simulink model "Assignment_acm"  (R2019b)
settings: Solver=VariableStepAuto  StartTime=0.0  StopTime=15.0  RelTol=1e-3
libraries: simulink x5, powerlib x4, eePowerMeasurement x1
settings Model: SnapshotBufferSize=20  SnapshotInterval=20  Creator=manda  LastModifiedBy=manda

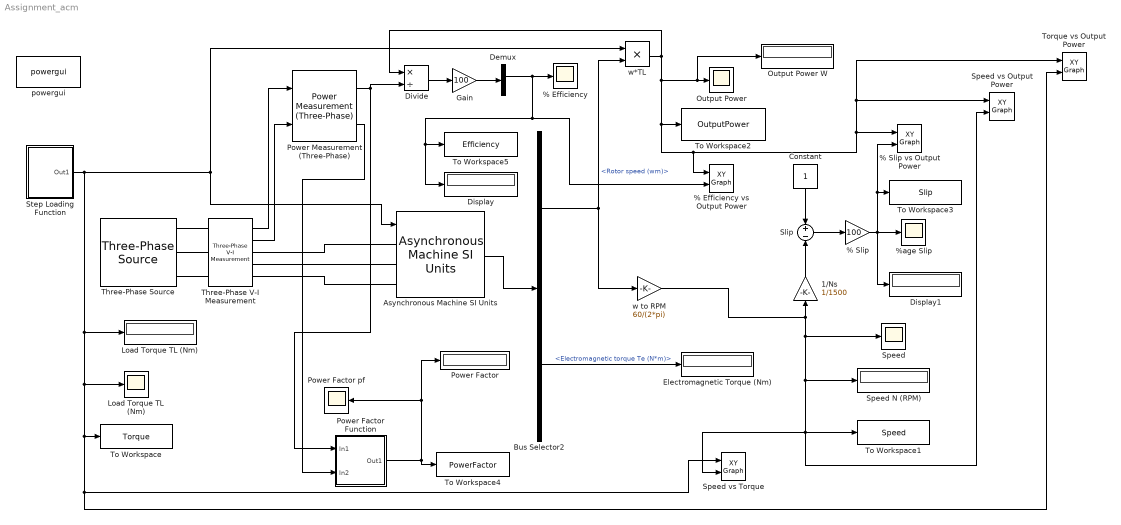
== system Assignment_acm ==
  % Efficiency : Scope
  % Efficiency vs Output Power : simulink/Sinks/XY Graph  xmin=0  xmax=inf  ymin=0  ymax=inf  st=0.1
  % Slip : Gain  Gain=100
  % Slip vs Output Power : simulink/Sinks/XY Graph  xmin=0  xmax=inf  ymin=0  ymax=inf  st=0.1
  %age Slip : Scope
  1/Ns : Gain  Gain=1/1500
  Asynchronous Machine SI Units : powerlib/Machines/Asynchronous Machine SI Units  RotorType=Squirrel-cage  PresetModel=No  MechanicalLoad=Torque Tm  ShowDetailedParameters=on  ReferenceFrame=Rotor  Units=SI  MeasurementBus=off  NominalParameters=[3700 415 50]  Stator=[1.405 0.005839]  Rotor=[1.395 0.005839]  Cage1=[0.4155 0.002066]  Cage2=[0.4168 0.0003495]  Lm=0.1722  Mechanical=[0.0131 0.002985 2]  PolePairs=2  InitialConditions=[0 0 0 0 0 0 0 0]  SimulateSaturation=off  Saturation=[14.03593122, 27.81365428, 53.79336849, 72.68890987, 97.98006896, 148.6815601, 215.7428561, 302.9841135, 428.7778367 ; 230, 322, 414, 460, 506, 552, 598, 644, 690]  LoadFlowParameters=1492000  TsPowergui=0  TsBlock=-1  IterativeModel=Trapezoidal non iterative  IterativeDiscreteModel=Trapezoidal non iterative  Pmec=1.492e+006
      settings: SourceProductName=Simscape Electrical
  Bus Selector2 : BusSelector  OutputSignals=Mechanical.Rotor speed (wm),Mechanical.Electromagnetic torque Te (N*m)
  Constant : Constant
  Demux : Demux
  Display : Display
  Display1 : Display
  Divide : Product  Inputs=*/
  Electromagnetic Torque (Nm) : Display
  Gain : Gain  Gain=100
  Load Torque TL (Nm) : Display
  "Load Torque TL (Nm) " : Scope
  Output Power : Scope
  Output Power W : Display
  Power Factor : Display
  Power Factor Function : Subsystem
  Power Factor pf : Scope
  Power Measurement (Three-Phase) : eePowerMeasurement/Power Measurement (Three-Phase)  LabelModeActiveChoice=Continuous  F=50  K=[0 1 2 3]  Seq=Positive  Ts=0
      settings: SourceProductName=Simscape Electrical  SourceProductBaseCode=PS
  Slip : Sum  Inputs=+-
  Speed : Scope
  Speed N (RPM) : Display
  Speed vs Output Power : simulink/Sinks/XY Graph  xmin=0  xmax=inf  ymin=0  ymax=inf  st=0.1
  Speed vs Torque : simulink/Sinks/XY Graph  xmin=0  xmax=inf  ymin=0  ymax=inf  st=0.1
  Step Loading Function : Subsystem
  Three-Phase V-I Measurement : powerlib/Measurements/Three-Phase V-I Measurement  VoltageMeasurement=phase-to-ground  SetLabelV=off  LabelV=Vabc  Vpu=off  VpuLL=off  CurrentMeasurement=yes  SetLabelI=off  LabelI=Iabc  Ipu=off  Pbase=100e6  Vbase=500e3  OutputType=Complex  PhasorSimulation=off  PSBequivalent=0
      settings: SourceProductName=Simscape Electrical
  Three-Phase Source : powerlib/Electrical Sources/Three-Phase Source  InternalConnection=Yg  VoltagePhases=off  Voltage=415  PhaseAngle=0  Voltage_phases=[25e3 25e3 25e3]/sqrt(3)  PhaseAngles_phases=[0 -120 +120]  Frequency=50  NonIdealSource=off  SpecifyImpedance=off  Resistance=0  Inductance=0  ShortCircuitLevel=100e6  BaseVoltage=25e3  XRratio=7  BusType=swing  Pref=10e3  Qref=0  Prefabc=[10e3, 10e3, 10e3]  Qrefabc=[0, 0, 0]  Qmin=-inf  Qmax=inf
      settings: SourceProductName=Simscape Electrical
  To Workspace : ToWorkspace  VariableName=Torque  SampleTime=0.1
      settings: Decimation=2
  To Workspace1 : ToWorkspace  VariableName=Speed  SampleTime=0.1
      settings: Decimation=2
  To Workspace2 : ToWorkspace  VariableName=OutputPower  SampleTime=0.1
      settings: Decimation=2
  To Workspace3 : ToWorkspace  VariableName=Slip  SampleTime=0.1
      settings: Decimation=2
  To Workspace4 : ToWorkspace  VariableName=PowerFactor  SampleTime=0.1
      settings: Decimation=2
  To Workspace5 : ToWorkspace  VariableName=Efficiency  SampleTime=0.1
      settings: Decimation=2
  Torque vs Output Power : simulink/Sinks/XY Graph  xmin=0  xmax=inf  ymin=0  ymax=inf  st=0.1
  powergui : powerlib/powergui  Priority=1  SimulationMode=Continuous  SampleTime=50e-6  frequency=60  Iterations=50  frequencyindice=50  Pbase=100e6  ErrMax=1e-4  UnitsV=kV  UnitsW=MW  buscounter=0  FunctionMessages=off  echomessages=off  EnableUseOfTLC=off  CurrentSourceSwitches=off  DisableSnubberDevices=off  DisableRonSwitches=off  DisableVfSwitches=off  DisplayEquations=off  AutomaticDiscreteSolvers=off  SolverType=Tustin/Backward Euler (TBE)  Interpol=off  ExternalGateDelay=off  methode=off  Ts=100  x0status=blocks  SPID=on  SwTol=0  HookPort=off  NonlinearTolerance=1e-4  nMaxIteration=100  ContinueOnMaxIteration=off  RestoreLinks=warning  ResistiveCurrentMeasurement=off  Frange=[0:2:500]  Ylog=off  Xlog=on  ShowGrid=off  save=off  variable=ZData  structure=0  ZoomFFT=off  StartTime=0.0  cycles=1  DisplayStyle=1  fundamental=60  FreqAxis=off  MaxFrequency=1000  frequencyindicesteady=1  RmsSteady=1  display=off
      settings: SourceProductName=Simscape Electrical
  w to RPM : Gain  Gain=60/(2*pi)
  w*TL : Product
  wires:
  Asynchronous Machine SI Units/1 -> Bus Selector2/1
  Bus Selector2/1 -> w*TL/2, w to RPM/1  "<Rotor speed (wm)>"
  Bus Selector2/2 -> Electromagnetic Torque (Nm)/1  "<Electromagnetic torque Te (N*m)>"
  w to RPM/1 -> Speed/1, Speed N (RPM)/1, To Workspace1/1, Speed vs Output Power/2, Speed vs Torque/2, 1/Ns/1
  Step Loading Function/1(Out1) -> Torque vs Output Power/2, Speed vs Torque/1, To Workspace/1, "Load Torque TL (Nm) "/1, Load Torque TL (Nm)/1, Asynchronous Machine SI Units/1, w*TL/1
  Constant/1 -> Slip/1
  1/Ns/1 -> Slip/2
  Slip/1 -> % Slip/1
  w*TL/1 -> Divide/1, % Efficiency vs Output Power/1, % Slip vs Output Power/1, Speed vs Output Power/1, Torque vs Output Power/1, To Workspace2/1, Output Power W/1, Output Power/1
  % Slip/1 -> Display1/1, %age Slip/1, % Slip vs Output Power/2, To Workspace3/1
  Power Measurement (Three-Phase)/1 -> Divide/2, Power Factor Function/1(In1)
  Power Measurement (Three-Phase)/2 -> Power Factor Function/2(In2)
  Power Factor Function/1(Out1) -> Power Factor pf/1, Power Factor/1, To Workspace4/1
  Three-Phase V-I Measurement/1 -> Power Measurement (Three-Phase)/1
  Three-Phase V-I Measurement/2 -> Power Measurement (Three-Phase)/2
  Divide/1 -> Gain/1
  Gain/1 -> Demux/1
  Demux/2 -> % Efficiency/1, % Efficiency vs Output Power/2, Display/1, To Workspace5/1
  connections:
  Three-Phase V-I Measurement/LConn1 -- Three-Phase Source/RConn1
  Three-Phase V-I Measurement/LConn2 -- Three-Phase Source/RConn2
  Three-Phase V-I Measurement/RConn1 -- Asynchronous Machine SI Units/LConn1
  Three-Phase V-I Measurement/RConn2 -- Asynchronous Machine SI Units/LConn2
  Three-Phase V-I Measurement/RConn3 -- Asynchronous Machine SI Units/LConn3
  Three-Phase V-I Measurement/LConn3 -- Three-Phase Source/RConn3

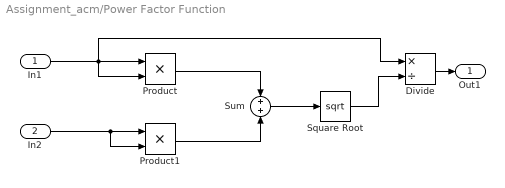
== system Assignment_acm/Power Factor Function ==
  In1 : Inport
  In2 : Inport  Port=2
  Divide : Product  Inputs=*/
  Product : Product
  Product1 : Product
  Square Root : Sqrt  SaturateOnIntegerOverflow=on
  Sum : Sum
  Out1 : Outport
  wires:
  Product1/1 -> Sum/2
  Product/1 -> Sum/1
  Sum/1 -> Square Root/1
  In2/1 -> Product1/2, Product1/1
  Square Root/1 -> Divide/2
  In1/1 -> Product/2, Divide/1, Product/1
  Divide/1 -> Out1/1

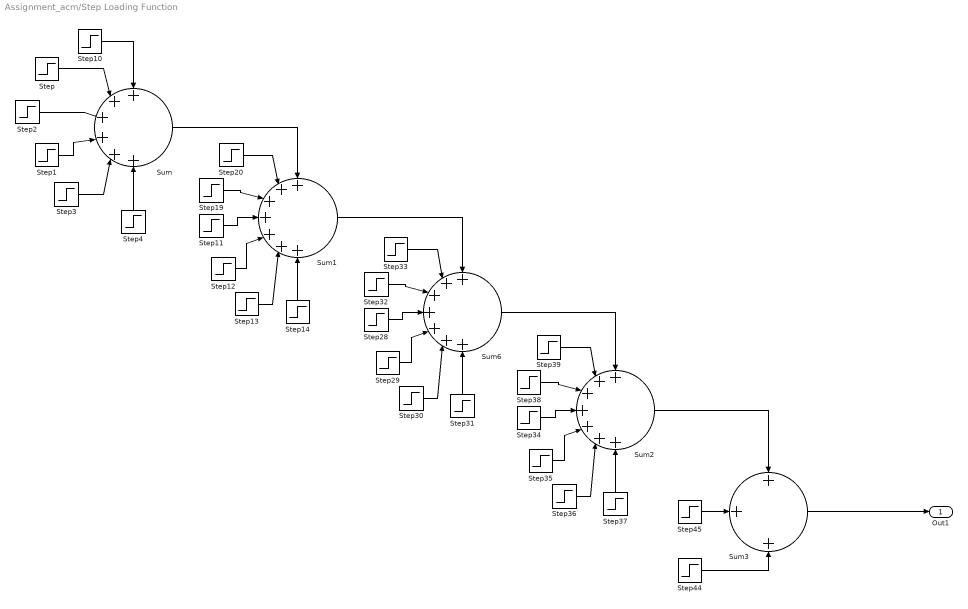
== system Assignment_acm/Step Loading Function ==
  Step : Step  Time=1.5  After=1.23  SampleTime=0
  Step1 : Step  Time=2.5  After=1.23  SampleTime=0
  Step10 : Step  After=1.23  SampleTime=0
  Step11 : Step  Time=5  After=1.23  SampleTime=0
  Step12 : Step  Time=5.5  After=1.23  SampleTime=0
  Step13 : Step  Time=6  After=1.23  SampleTime=0
  Step14 : Step  Time=6.5  After=1.23  SampleTime=0
  Step19 : Step  Time=4.5  After=1.23  SampleTime=0
  Step2 : Step  Time=2  After=1.23  SampleTime=0
  Step20 : Step  Time=4  After=1.23  SampleTime=0
  Step28 : Step  Time=8  After=1.23  SampleTime=0
  Step29 : Step  Time=8.5  After=1.23  SampleTime=0
  Step3 : Step  Time=3  After=1.23  SampleTime=0
  Step30 : Step  Time=9  After=1.23  SampleTime=0
  Step31 : Step  Time=9.5  After=1.23  SampleTime=0
  Step32 : Step  Time=7.5  After=1.23  SampleTime=0
  Step33 : Step  Time=7  After=1.23  SampleTime=0
  Step34 : Step  Time=11  After=1.23  SampleTime=0
  Step35 : Step  Time=11.5  After=1.23  SampleTime=0
  Step36 : Step  Time=12  After=1.23  SampleTime=0
  Step37 : Step  Time=12.5  After=1.23  SampleTime=0
  Step38 : Step  Time=10.5  After=1.23  SampleTime=0
  Step39 : Step  Time=10  After=1.23  SampleTime=0
  Step4 : Step  Time=3.5  After=1.23  SampleTime=0
  Step44 : Step  Time=13.5  After=1.23  SampleTime=0
  Step45 : Step  Time=13  After=1.23  SampleTime=0
  Sum : Sum  Inputs=6
  Sum1 : Sum  Inputs=7
  Sum2 : Sum  Inputs=7
  Sum3 : Sum  Inputs=3
  Sum6 : Sum  Inputs=7
  Out1 : Outport
  wires:
  Step34/1 -> Sum2/4
  Step12/1 -> Sum1/5
  Step36/1 -> Sum2/6
  Step37/1 -> Sum2/7
  Step30/1 -> Sum6/6
  Step13/1 -> Sum1/6
  Step2/1 -> Sum/3
  Sum/1 -> Sum1/1
  Step3/1 -> Sum/5
  Sum6/1 -> Sum2/1
  Step31/1 -> Sum6/7
  Step35/1 -> Sum2/5
  Step38/1 -> Sum2/3
  Sum2/1 -> Sum3/1
  Step29/1 -> Sum6/5
  Step39/1 -> Sum2/2
  Step1/1 -> Sum/4
  Step28/1 -> Sum6/4
  Sum1/1 -> Sum6/1
  Step20/1 -> Sum1/2
  Step11/1 -> Sum1/4
  Step/1 -> Sum/2
  Step4/1 -> Sum/6
  Step19/1 -> Sum1/3
  Step10/1 -> Sum/1
  Step45/1 -> Sum3/2
  Step44/1 -> Sum3/3
  Step14/1 -> Sum1/7
  Step33/1 -> Sum6/2
  Step32/1 -> Sum6/3
  Sum3/1 -> Out1/1
